simulink model "simulink6step"  (R2021b)
settings: Solver=FixedStepAuto  StartTime=0.0  StopTime=0.01  FixedStep=5e-7  RelTol=1e-3
libraries: spsIGBTDiodeLib x6, spsCurrentMeasurementLib x3, spsSeriesRLCBranchLib x3, simulink x2, spsDCVoltageSourceLib x1, spsGroundLib x1, spspowerguiLib x1
settings Model: Creator=eeysh5  LastModifiedBy=Sam

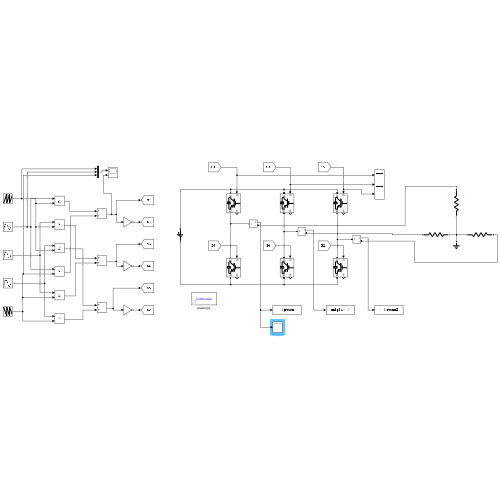
[thumbnail: Simulink's stored preview of the top-level diagram]
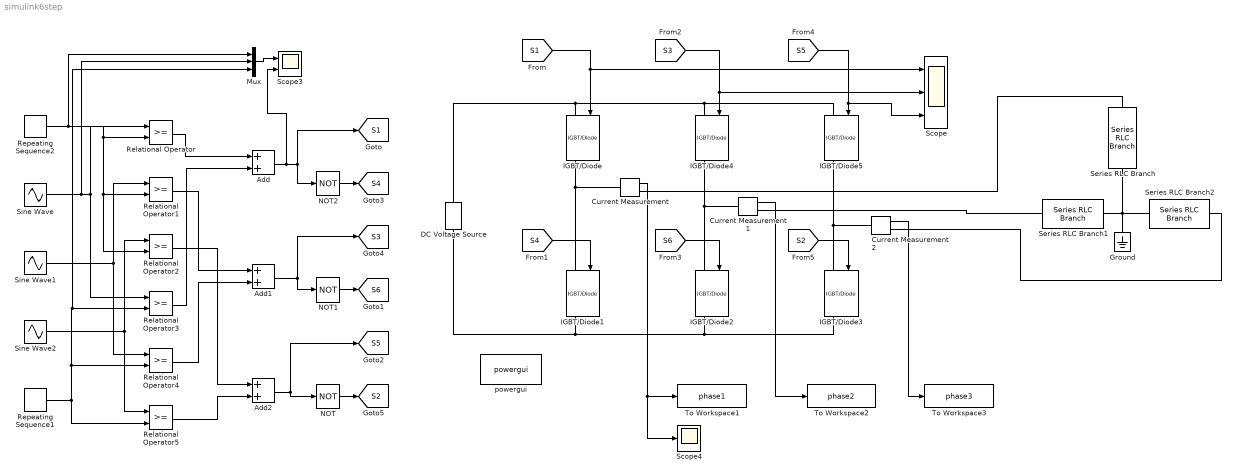
== system simulink6step ==
  Add : Sum
  Add1 : Sum
  Add2 : Sum
  Current Measurement : spsCurrentMeasurementLib/Current Measurement  PhasorSimulation=off  OutputType=Complex  PSBequivalent=0
  Current Measurement1 : spsCurrentMeasurementLib/Current Measurement  PhasorSimulation=off  OutputType=Complex  PSBequivalent=0
  Current Measurement2 : spsCurrentMeasurementLib/Current Measurement  PhasorSimulation=off  OutputType=Complex  PSBequivalent=0
  DC Voltage Source : spsDCVoltageSourceLib/DC Voltage Source  Amplitude=5687  Measurements=None
  Ground : spsGroundLib/Ground  LConnTagsString=a
  IGBT/Diode{,1..5} (6 alike) : spsIGBTDiodeLib/IGBT//Diode  Ron=1e-3  Rs=1e5  Cs=inf  Measurements=on
  Mux : Mux  Inputs=3
  NOT : Logic  Operator=NOT  IconShape=distinctive  AllPortsSameDT=off  OutDataTypeStr=boolean
  NOT1 : Logic  Operator=NOT  IconShape=distinctive  AllPortsSameDT=off  OutDataTypeStr=boolean
  NOT2 : Logic  Operator=NOT  IconShape=distinctive  AllPortsSameDT=off  OutDataTypeStr=boolean
  Relational Operator{,1..5} (6 alike) : RelationalOperator  OutDataTypeStr=boolean  RndMeth=Simplest
  Repeating Sequence1 : simulink/Sources/Repeating Sequence  rep_seq_t=[0 1e-5]  rep_seq_y=[0 -1]
  Repeating Sequence2 : simulink/Sources/Repeating Sequence  rep_seq_t=[0 1e-5]  rep_seq_y=[0 1]
  Scope : Scope  NumInputPorts=3
  Scope3 : Scope  NumInputPorts=2
  Scope4 : Scope
  Series RLC Branch : spsSeriesRLCBranchLib/Series RLC Branch  LConnTagsString=__new0  RConnTagsString=__new0  BranchType=R  Resistance=1  Inductance=1e-3  SetiL0=off  InitialCurrent=0  Capacitance=1e-6  Setx0=off  InitialVoltage=0  Measurements=None
  Series RLC Branch1 : spsSeriesRLCBranchLib/Series RLC Branch  LConnTagsString=__new0  RConnTagsString=__new0  BranchType=R  Resistance=1  Inductance=1e-3  SetiL0=off  InitialCurrent=0  Capacitance=1e-6  Setx0=off  InitialVoltage=0  Measurements=None
  Series RLC Branch2 : spsSeriesRLCBranchLib/Series RLC Branch  LConnTagsString=__new0  RConnTagsString=__new0  BranchType=R  Resistance=1  Inductance=1e-3  SetiL0=off  InitialCurrent=0  Capacitance=1e-6  Setx0=off  InitialVoltage=0  Measurements=None
  Sine Wave : Sin  Frequency=2*pi*2000  SampleTime=0
  Sine Wave1 : Sin  Frequency=2*pi*2000  Phase=(2*pi)/3  SampleTime=0
  Sine Wave2 : Sin  Frequency=2*pi*2000  Phase=(4*pi)/3  SampleTime=0
  To Workspace1 : ToWorkspace  VariableName=phase1  SaveFormat=Timeseries  SampleTime=-1
  To Workspace2 : ToWorkspace  VariableName=phase2  SaveFormat=Timeseries  SampleTime=-1
  To Workspace3 : ToWorkspace  VariableName=phase3  SaveFormat=Timeseries  SampleTime=-1
  powergui : spspowerguiLib/powergui  Priority=1  SimulationMode=Continuous  SampleTime=50e-6  frequency=60  Iterations=50  frequencyindice=0  Pbase=1e6  ErrMax=1e-4  UnitsV=kV  UnitsW=MW  buscounter=0  FunctionMessages=off  echomessages=off  EnableUseOfTLC=off  CurrentSourceSwitches=off  DisableSnubberDevices=off  DisableRonSwitches=off  DisableVfSwitches=off  DisplayEquations=off  AutomaticDiscreteSolvers=off  SolverType=Tustin/Backward Euler (TBE)  Interpol=off  ExternalGateDelay=off  methode=off  Ts=100  x0status=blocks  SPID=on  SwTol=0  HookPort=off  NonlinearTolerance=1e-4  nMaxIteration=100  ContinueOnMaxIteration=off  RestoreLinks=warning  ResistiveCurrentMeasurement=off  Frange=[0:2:500]  Ylog=off  Xlog=on  ShowGrid=off  save=off  variable=ZData  structure=0  ZoomFFT=off  StartTime=0.0  cycles=1  DisplayStyle=1  fundamental=60  FreqAxis=off  MaxFrequency=1000  frequencyindicesteady=1  RmsSteady=1  display=off
  tag scope: S1=global, S2=global, S3=global, S4=global, S5=global, S6=global
  wires:
  NOT2/1 -> [S4]
  NOT1/1 -> [S6]
  NOT/1 -> [S2]
  [S1] -> IGBT/Diode/1, Scope/1
  [S3] -> IGBT/Diode4/1, Scope/2
  [S4] -> IGBT/Diode1/1
  [S6] -> IGBT/Diode2/1
  [S2] -> IGBT/Diode3/1
  [S5] -> Scope/3, IGBT/Diode5/1
  Repeating Sequence2/1 -> Mux/1, Relational Operator/2, Relational Operator1/2, Relational Operator2/2
  Sine Wave/1 -> Mux/2, Relational Operator/1, Relational Operator3/1
  Sine Wave1/1 -> Relational Operator1/1, Relational Operator4/1
  Sine Wave2/1 -> Relational Operator2/1, Relational Operator5/1
  Repeating Sequence1/1 -> Relational Operator5/2, Relational Operator4/2, Mux/3, Relational Operator3/2
  Relational Operator/1 -> Add/1
  Relational Operator3/1 -> Add/2
  Relational Operator4/1 -> Add1/2
  Relational Operator1/1 -> Add1/1
  Relational Operator2/1 -> Add2/1
  Relational Operator5/1 -> Add2/2
  Add1/1 -> [S3], NOT1/1
  Add2/1 -> [S5], NOT/1
  Add/1 -> Scope3/2, [S1], NOT2/1
  Mux/1 -> Scope3/1
  Current Measurement/1 -> Scope4/1, To Workspace1/1
  Current Measurement1/1 -> To Workspace2/1
  Current Measurement2/1 -> To Workspace3/1
  connections:
  IGBT/Diode/RConn1 -- IGBT/Diode1/LConn1 -- Current Measurement/LConn1
  IGBT/Diode4/RConn1 -- IGBT/Diode2/LConn1 -- Current Measurement1/LConn1
  IGBT/Diode5/RConn1 -- Current Measurement2/LConn1 -- IGBT/Diode3/LConn1
  DC Voltage Source/RConn1 -- IGBT/Diode/LConn1 -- IGBT/Diode4/LConn1 -- IGBT/Diode5/LConn1
  IGBT/Diode3/RConn1 -- IGBT/Diode2/RConn1 -- IGBT/Diode1/RConn1 -- DC Voltage Source/LConn1
  Series RLC Branch/LConn1 -- Current Measurement/RConn1
  Series RLC Branch1/LConn1 -- Current Measurement1/RConn1
  Series RLC Branch2/LConn1 -- Current Measurement2/RConn1
  Series RLC Branch1/RConn1 -- Ground/LConn1 -- Series RLC Branch2/RConn1 -- Series RLC Branch/RConn1
